simulink model "Slave_Env_PD"  (R2020a)
settings: Solver=VariableStepAuto  StartTime=0.0  StopTime=10  RelTol=1e-3
values from neighbouring files (symbols this model uses):
  Be = 5    [Teleop_parameters.m]    (also in base.mat = 0.5; base_no_attrito.mat = 0.5; ci_siamo.mat; force_control.mat = 0.5)
  k_s = 19.34    [Teleop_parameters.m]    (also in base.mat; base_no_attrito.mat; ci_siamo.mat; force_control.mat)
  Kc2v_s = 2    [Teleop_parameters.m]    (also in base.mat; base_no_attrito.mat; ci_siamo.mat; force_control.mat)
  Ke = 10    [Teleop_parameters.m]    (also in base.mat; base_no_attrito.mat; ci_siamo.mat; force_control.mat)
  Kt2c_s = 1.182    [Teleop_parameters.m]    (also in base.mat; base_no_attrito.mat; ci_siamo.mat; force_control.mat)
  lArm_s = 0.1    [Teleop_parameters.m]    (also in base.mat; base_no_attrito.mat; ci_siamo.mat; force_control.mat)
  maxCurrent_s = 4.5    [Teleop_parameters.m]    (also in base.mat; base_no_attrito.mat; ci_siamo.mat; force_control.mat)
  qe = 10    [Teleop_parameters.m]    (also in base.mat = 5; base_no_attrito.mat = 5; ci_siamo.mat = 0.5; force_control.mat = 5)
  tau_s = 1.217    [Teleop_parameters.m]    (also in base.mat; base_no_attrito.mat; ci_siamo.mat; force_control.mat)
settings Model: Creator=riccardo  LastModifiedBy=gbagolin

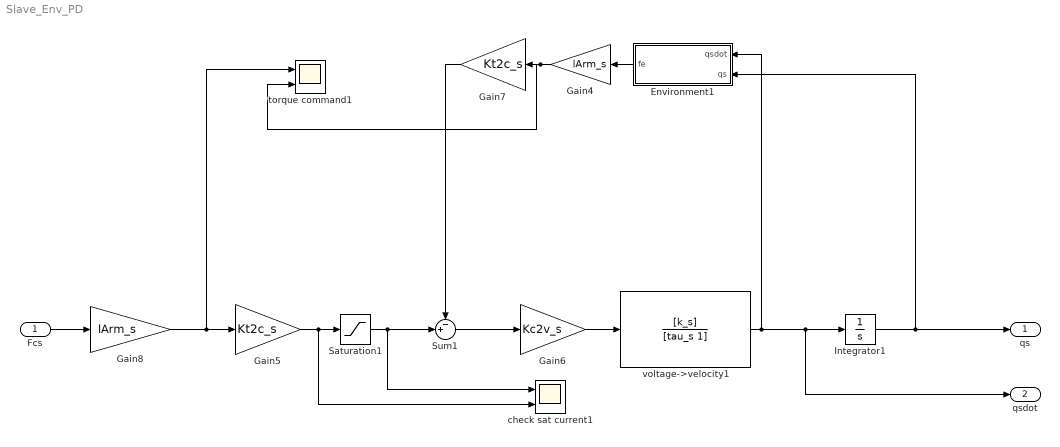
== system Slave_Env_PD ==
  Fcs : Inport
  Environment1 : Subsystem
  Gain4 : Gain  Gain=lArm_s
  Gain5 : Gain  Gain=Kt2c_s
  Gain6 : Gain  Gain=Kc2v_s
  Gain7 : Gain  Gain=Kt2c_s
  Gain8 : Gain  Gain=lArm_s
  Integrator1 : Integrator
  Saturation1 : Saturate  UpperLimit=maxCurrent_s  LowerLimit=-maxCurrent_s
  Sum1 : Sum  Inputs=-+|
  check sat current1 : Scope  NumInputPorts=2
  torque command1 : Scope  NumInputPorts=2
  voltage->velocity1 : TransferFcn  Numerator=[k_s]  Denominator=[tau_s 1]
  qs : Outport
  qsdot : Outport  Port=2
  wires:
  Sum1/1 -> Gain6/1
  Gain4/1 -> torque command1/2, Gain7/1
  Environment1/1(fe) -> Gain4/1
  voltage->velocity1/1 -> Environment1/1(qsdot), qsdot/1, Integrator1/1
  Gain8/1 -> torque command1/1, Gain5/1
  Fcs/1 -> Gain8/1
  Saturation1/1 -> Sum1/2, check sat current1/1
  Gain7/1 -> Sum1/1
  Gain6/1 -> voltage->velocity1/1
  Integrator1/1 -> qs/1, Environment1/2(qs)
  Gain5/1 -> check sat current1/2, Saturation1/1

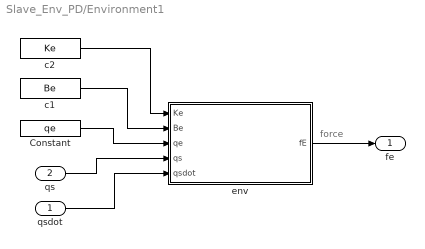
== system Slave_Env_PD/Environment1 ==
  note: force
  qsdot : Inport
  qs : Inport  Port=2
  Constant : Constant  Value=qe  SampleTime=0
  c1 : Constant  Value=Be  SampleTime=0
  c2 : Constant  Value=Ke  SampleTime=0
  env : MATLAB Function  TreatAsAtomicUnit=on
  fe : Outport  VectorParamsAs1DForOutWhenUnconnected=off
  wires:
  Constant/1 -> env/3(qe)
  c1/1 -> env/2(Be)
  c2/1 -> env/1(Ke)
  qs/1 -> env/4(qs)
  qsdot/1 -> env/5(qsdot)
  env/1(fE) -> fe/1

== matlab function Slave_Env_PD/Environment1/env ==
  data: Ke input; Be input; qe input; qs input; fE output; qsdot input
function fE  = environment(Ke, Be, qe, qs, qsdot)
if qs > qe
   fE = Ke * (qs - qe) + Be * qsdot;
else
   fE = 0;
end
